simulink model "rec_shape (1)"  (R2023b)
settings: Solver=VariableStepAuto  StartTime=0.0  StopTime=10.0  RelTol=1e-3
undefined symbols (not defined in the file): gray
libraries: visionsources x1
settings Model: Creator=DELL  LastModifiedBy=DELL
settings DebuggingCC: UnderSpecifiedDimensionMsg=warning

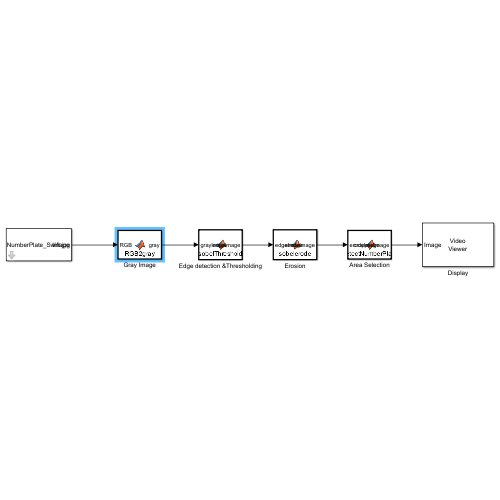
[thumbnail: Simulink's stored preview of the top-level diagram]
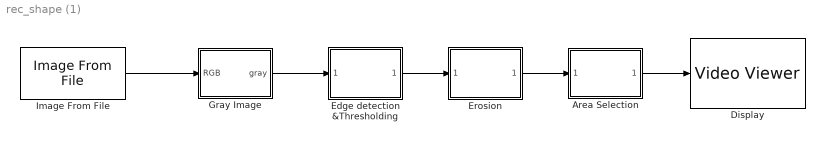
== system rec_shape (1) ==
  Area Selection : MATLAB Function  TreatAsAtomicUnit=on
  Display : VideoViewer  colormapValue=gray(256)  FigPos=[1 814 1536 716]
  Edge detection &Thresholding : MATLAB Function  TreatAsAtomicUnit=on
  Erosion : MATLAB Function  TreatAsAtomicUnit=on
  Gray Image : MATLAB Function  TreatAsAtomicUnit=on
  Image From File : visionsources/Image From File  Tag=vipblks_nd  FileName=C:\Users\DELL\Downloads\NumberPlate_Swift.jpg  Ts=inf  imagePorts=One multidimensional signal  OutPortLabels=R|G|B  ImageDataType=Inherit from input image  sdImageDataType=uint(8)  Signed=on  WordLength=16  FractionLengthMode=User-defined  FractionLength=15
  wires:
  Image From File/1 -> Gray Image/1(RGB)
  Gray Image/1(gray) -> Edge detection &Thresholding/1(grayImage)
  Edge detection &Thresholding/1(edgeImage) -> Erosion/1(edgeImage)
  Erosion/1(erodeImage) -> Area Selection/1(erodeImage)
  Area Selection/1(croppedImage) -> Display/1

== matlab function rec_shape (1)/Edge detection &Thresholding ==
  data: grayImage input; edgeImage output
function edgeImage = sobelThreshold(grayImage)
    % Sobel kernels
    k_horizontal = [-1 0 1; -2 0 2; -1 0 1];
    k_vertical = [-1 -2 -1; 0 0 0; 1 2 1];

    % Calculate horizontal and vertical gradients
    H = conv2(double(grayImage), k_horizontal, 'same');
    V = conv2(double(grayImage), k_vertical, 'same');

    E = sqrt(H.^2 + V.^2);

    E = E / max(E(:));

    threshold = 0.4;
    edgeImage = E > threshold;
end

== matlab function rec_shape (1)/Erosion ==
  data: edgeImage input; erodeImage output
function erodeImage = sobelerode(edgeImage)
    SE = strel('square', 1);
    erodeImage = imerode(edgeImage, SE);
    
end

== matlab function rec_shape (1)/Area Selection ==
  data: erodeImage input; croppedImage output
function croppedImage = detectNumberPlate(erodeImage)
   
    [rows, cols, ~] = size(erodeImage);  

    x = round(cols/4);        
    y = round(rows/2);        
    width = min(450, cols/2); 
    height = min(200, rows/4); 

    croppedImage = imcrop(erodeImage, [x, y, width-1, height-1]);
end

== matlab function rec_shape (1)/Gray Image ==
  data: RGB input; gray output
function gray = RGB2gray(RGB)
    gray = rgb2gray(RGB);
end
